simulink model "LF_AC29bus_HVDCdemo_V2_1"  (R2019b)
settings: Solver=FixedStepDiscrete  StartTime=0.0  StopTime=fix(6/Ts)*Ts  FixedStep=Ts  RelTol=1e-3
InitFcn:
  | Ts_avg=150e-6;
  | Ts=50e-6;
  | 
  | %Tc_stab = 1/60/5;
  | %Tc_stab = 2/60;
  | Tc_stab = Ts;
  | 
  | 
  | Ts_avg=150e-6;
  | 
  | Ts=50e-6;
  | 
  | % Rectifier AC side :
  | VLL_nom_R = 735e3; % V
  | Fnom_R = 60;           % Hz
  | 
  | % Inverter AC side :
  | VLL_nom_I = 735e3; % V
  | Fnom_I = 60;           % Hz
  | 
  | % DC :
  | Vdc_nom = 500e3;   % V
  | Idc_nom  = 2000;     % A
undefined symbols (not defined in the file): D1, D11, Delta, test_alpha
libraries: powerlib x223, powerlib_meascontrol x57, simulink x22, sps_avr x7
(part 10 of 10)

== system LF_AC29bus_HVDCdemo_V2_1/HVDC_network_avg/Rectifier Control and Protection (Average model)/Rectifier Pole Control (Current)/Gamma Regulator/PI Regulator with external limits and linrarized Kp (Discrete)1/S16 ==
  note: INTEGRATOR with External limits & Reset & Hold
  note: Gain * Ts
  Max : Inport
  Min : Inport  Port=2
  In : Inport  Port=3
  Reset : Inport  Port=4
  Hold : Inport  Port=5
  Reset Value : Inport  Port=6
  Gain1 : Gain  Gain=k*st  SaturateOnIntegerOverflow=on  OutDataTypeStr=Inherit: Same as input  ParamDataTypeStr=Inherit: Same as input
  IC = ic : UnitDelay  InitialCondition=ic  SampleTime=st  HasFrameUpgradeWarning=on
  Logical Operator4 : Logic  Operator=OR
  MinMax : MinMax  Inputs=2  SaturateOnIntegerOverflow=on  InputSameDT=on
  MinMax1 : MinMax  Function=max  Inputs=2  SaturateOnIntegerOverflow=on  InputSameDT=on
  Saturation Dynamic : simulink/Discontinuities/Saturation Dynamic  OutMin=[]  OutMax=[]  OutDataTypeStr=Inherit: Same as second input  OutDataType=fixdt(1, 16)  OutScaling=2^-10  DoSatur=off
  Sum : Sum  SaturateOnIntegerOverflow=on  InputSameDT=on  OutDataTypeStr=Inherit: Same as first input
  Switch2 : Switch  Criteria=u2 > Threshold  SaturateOnIntegerOverflow=on  InputSameDT=on
  Switch3 : Switch  Criteria=u2 > Threshold  SaturateOnIntegerOverflow=on  InputSameDT=on
  Switch7 : Switch  Criteria=u2 > Threshold  SaturateOnIntegerOverflow=on  InputSameDT=on
  Out : Outport  InitialOutput=0
  wires:
  Saturation Dynamic/1 -> Out/1, IC = ic/1
  Gain1/1 -> Sum/1
  In/1 -> Gain1/1
  Sum/1 -> Saturation Dynamic/2
  Hold/1 -> Logical Operator4/1
  Reset/1 -> Switch7/2, Logical Operator4/2
  Logical Operator4/1 -> Switch2/2, Switch3/2
  Switch2/1 -> MinMax/1
  Max/1 -> Switch2/3, MinMax/2
  Reset Value/1 -> Switch7/1
  MinMax/1 -> Saturation Dynamic/1
  MinMax1/1 -> Saturation Dynamic/3
  Switch3/1 -> MinMax1/1
  Min/1 -> Switch3/3, MinMax1/2
  IC = ic/1 -> Switch7/3
  Switch7/1 -> Switch3/1, Sum/2, Switch2/1

== system LF_AC29bus_HVDCdemo_V2_1/HVDC_network_avg/Rectifier Control and Protection (Average model)/Rectifier Pole Control (Current)/Voltage Regulator/PI Regulator with external limits and linrarized Kp (Discrete)/Kp Linearisation ==
  note: Kp Linearization
  Alpha_lin : Inport
  Kp : Inport  Port=2
  Inv : Inport  Port=3
  Min_lin : Inport  Port=4
  Max_lin : Inport  Port=5
  Constant3 : Constant  Value=On_lin
  Data Type Conversion : DataTypeConversion  OutDataTypeStr=boolean  SaturateOnIntegerOverflow=on  RndMeth=Zero
  Logical Operator : Logic  Operator=NOT
  Logical Operator1 : Logic  Operator=NOT
  Math Function : Math  Operator=reciprocal  SaturateOnIntegerOverflow=on
  Prod2 : Product  Inputs=3  SaturateOnIntegerOverflow=on  InputSameDT=on  OutDataTypeStr=Inherit: Same as first input
  Saturation Dynamic : simulink/Discontinuities/Saturation Dynamic  OutMin=[]  OutMax=[]  OutDataTypeStr=Inherit: Same as second input  OutDataType=fixdt(1, 16)  OutScaling=2^-10  DoSatur=off
  Switch : Switch  Criteria=u2 > Threshold  SaturateOnIntegerOverflow=on  InputSameDT=on
  Switch1 : Switch  Criteria=u2 > Threshold  SaturateOnIntegerOverflow=on  InputSameDT=on
  Trigonometric Function : Trigonometry
  Trigonometric Function1 : Trigonometry
  k : Gain  Gain=pi/180  SaturateOnIntegerOverflow=on  OutDataTypeStr=Inherit: Same as input  ParamDataTypeStr=Inherit: Same as input
  k1 : Gain  Gain=pi/180  SaturateOnIntegerOverflow=on  OutDataTypeStr=Inherit: Same as input  ParamDataTypeStr=Inherit: Same as input
  Kp_lin : Outport  InitialOutput=0
  wires:
  Min_lin/1 -> Switch/1, Saturation Dynamic/3
  Max_lin/1 -> Saturation Dynamic/1, Switch/3
  Alpha_lin/1 -> Saturation Dynamic/2
  Math Function/1 -> Prod2/2
  Trigonometric Function1/1 -> Math Function/1
  k/1 -> Trigonometric Function1/1
  Kp/1 -> Switch1/1, Prod2/3
  Inv/1 -> Logical Operator/1
  Logical Operator/1 -> Switch/2
  Trigonometric Function/1 -> Prod2/1
  Saturation Dynamic/1 -> k/1
  k1/1 -> Trigonometric Function/1
  Switch/1 -> k1/1
  Switch1/1 -> Kp_lin/1
  Prod2/1 -> Switch1/3
  Logical Operator1/1 -> Switch1/2  "off"
  Constant3/1 -> Data Type Conversion/1
  Data Type Conversion/1 -> Logical Operator1/1

== system LF_AC29bus_HVDCdemo_V2_1/HVDC_network_avg/Rectifier Control and Protection (Average model)/Rectifier Pole Control (Current)/Voltage Regulator/PI Regulator with external limits and linrarized Kp (Discrete)/S16 ==
  note: INTEGRATOR with External limits & Reset & Hold
  note: Gain * Ts
  Max : Inport
  Min : Inport  Port=2
  In : Inport  Port=3
  Reset : Inport  Port=4
  Hold : Inport  Port=5
  Reset Value : Inport  Port=6
  Gain1 : Gain  Gain=k*st  SaturateOnIntegerOverflow=on  OutDataTypeStr=Inherit: Same as input  ParamDataTypeStr=Inherit: Same as input
  IC = ic : UnitDelay  InitialCondition=ic  SampleTime=st  HasFrameUpgradeWarning=on
  Logical Operator4 : Logic  Operator=OR
  MinMax : MinMax  Inputs=2  SaturateOnIntegerOverflow=on  InputSameDT=on
  MinMax1 : MinMax  Function=max  Inputs=2  SaturateOnIntegerOverflow=on  InputSameDT=on
  Saturation Dynamic : simulink/Discontinuities/Saturation Dynamic  OutMin=[]  OutMax=[]  OutDataTypeStr=Inherit: Same as second input  OutDataType=fixdt(1, 16)  OutScaling=2^-10  DoSatur=off
  Sum : Sum  SaturateOnIntegerOverflow=on  InputSameDT=on  OutDataTypeStr=Inherit: Same as first input
  Switch2 : Switch  Criteria=u2 > Threshold  SaturateOnIntegerOverflow=on  InputSameDT=on
  Switch3 : Switch  Criteria=u2 > Threshold  SaturateOnIntegerOverflow=on  InputSameDT=on
  Switch7 : Switch  Criteria=u2 > Threshold  SaturateOnIntegerOverflow=on  InputSameDT=on
  Out : Outport  InitialOutput=0
  wires:
  Saturation Dynamic/1 -> Out/1, IC = ic/1
  Gain1/1 -> Sum/1
  In/1 -> Gain1/1
  Sum/1 -> Saturation Dynamic/2
  Hold/1 -> Logical Operator4/1
  Reset/1 -> Switch7/2, Logical Operator4/2
  Logical Operator4/1 -> Switch2/2, Switch3/2
  Switch2/1 -> MinMax/1
  Max/1 -> Switch2/3, MinMax/2
  Reset Value/1 -> Switch7/1
  MinMax/1 -> Saturation Dynamic/1
  MinMax1/1 -> Saturation Dynamic/3
  Switch3/1 -> MinMax1/1
  Min/1 -> Switch3/3, MinMax1/2
  IC = ic/1 -> Switch7/3
  Switch7/1 -> Switch3/1, Sum/2, Switch2/1

== matlab function LF_AC29bus_HVDCdemo_V2_1/HVDC_network_avg/Inverter Average model/HVDC_CONV_AVG/Average Model Computation/DC_AVG_EQ MATLAB Function ==
  data: Ud output; alpha_deg input; Tap_pu input; Id input; I_dq output; Udi0 input; w input; Lc parameter size=1; m output; R12 parameter size=1; Vf parameter size=1; Ron parameter size=1; Ratio_nom parameter size=1
% Embedded function : DC_AVG_EQ
% By: Silvano Casoria (Hydro-Queec)
% Date: January 2011, December 2012
% Description: Implement the equations of the average model of an HVDC
%              converter unit (transformer and 6 pulse bridge).
% 
%
function [Ud,I_dq, m]=DC_AVG_EQ(alpha_deg,Tap_pu,Id,Udi0,w,...
Lc, R12, Vf, Ron, Ratio_nom)
%
% INPUTS:
% alpha_deg: Firing angle from the control system (deg)
% Tap_pu: Per-unit tap ratio (Npripary/Nsecondary)
% Id:   DC current (A)
% Udi0: Ideal no load direct voltage (V)
% w:    System angular frequency (rad/s)
%
% OUTPUTS:
% Ud: Direct voltage (V)
% I_dq: Two element vector [I_d, I_q] with I_d = d axis component of the
%       fondamental primary phase current, I_q = q axis componenet.
% m : Four element vector to measure internal variables.
%
% PARAMETERS (for one 6p bridge. Calculated in the model mask):
% Lc  = Commutation inductance, seen from the secondary (H)
% R12 = Total transformer resistance, seen from the secondary (ohm)
% Vf  = Thristor/Diode forward voltage (V)
% Ron = Thristor/Diode On resistance (ohm)
% Ratio_nom = Nominal transformer ratio (Uprim/Usec)

% Initialisation and declaration:
m = [0 0 0 0];

% Xc calculation :
Xc = Lc * w;

% Intermediary calculation :
Rc = Xc * 3/pi;              % Commutation resistance Rc (ohm)
Cos_alpha = cosd(alpha_deg); % (rad)
 
% Overlap angle calculation :
mu_deg = acosd( LIM((Cos_alpha-2*(Rc*Id/LIM(Udi0,eps,1e6))),-1,1) )- ...
         alpha_deg;  %(deg)
mu  = mu_deg*1.745329e-2;    % (rad)

% Exctinctoin angle (gamma_deg) deduction :
gamma_deg = 180 - alpha_deg - mu_deg;

% Transformer windings & Thyristor resistance drop Mean value
% a functoin of the commutation interval:
Req      = (2 - mu_deg/120) * (R12+Ron);
Req_drop = Req * Id;

% Thyristors forward drop:
Thy_drop = 2*Vf;

% Ud calculation :
Ud  = Udi0 * Cos_alpha - Rc*Id - Req_drop - Thy_drop;

% Fondamental primary phase current Ia1 components d and q axis 
% (Ia1 = I_d + j*I_q) (rms values):
Den = (Tap_pu*Ratio_nom*Xc*4*sqrt(6));
I_d = Udi0*(cosd(2*alpha_deg)-cosd(2*mu_deg+2*alpha_deg))/Den;
I_q = -Udi0*(2*mu+sind(2*alpha_deg) - sind(2*mu_deg+2*alpha_deg))/Den;
I_dq = [I_d, I_q]';
   
% Reactive power consumption (always positive):
Q = -(I_q*Udi0*pi*Ratio_nom*Tap_pu)/sqrt(6);  % (var)

% Active AC power flowing into the converter transformer :
P = (I_d*Udi0*pi*Ratio_nom*Tap_pu)/sqrt(6);   % (W)

% Measurements:
m(1) = Q;
m(2) = mu_deg;
m(3) = gamma_deg;
m(4) = P;

% ----------
function [Y_lim] = LIM(Y,Min,Max)
% Description : The output is the input signal limited between the
%               values Min and Max ([Min,Max]).
if (Y >= Max)
    Y_lim = Max;
elseif (Y <= Min)
    Y_lim = Min;
else
    Y_lim = Y;
end
% ======================= E N D ===============================

== matlab function LF_AC29bus_HVDCdemo_V2_1/HVDC_network_avg/Rectifier Average model/HVDC_CONV_AVG/Average Model Computation/DC_AVG_EQ MATLAB Function ==
  data: Ud output; alpha_deg input; Tap_pu input; Id input; I_dq output; Udi0 input; w input; Lc parameter size=1; m output; R12 parameter size=1; Vf parameter size=1; Ron parameter size=1; Ratio_nom parameter size=1
% Embedded function : DC_AVG_EQ
% By: Silvano Casoria (Hydro-Queec)
% Date: January 2011, December 2012
% Description: Implement the equations of the average model of an HVDC
%              converter unit (transformer and 6 pulse bridge).
% 
%
function [Ud,I_dq, m]=DC_AVG_EQ(alpha_deg,Tap_pu,Id,Udi0,w,...
Lc, R12, Vf, Ron, Ratio_nom)
%
% INPUTS:
% alpha_deg: Firing angle from the control system (deg)
% Tap_pu: Per-unit tap ratio (Npripary/Nsecondary)
% Id:   DC current (A)
% Udi0: Ideal no load direct voltage (V)
% w:    System angular frequency (rad/s)
%
% OUTPUTS:
% Ud: Direct voltage (V)
% I_dq: Two element vector [I_d, I_q] with I_d = d axis component of the
%       fondamental primary phase current, I_q = q axis componenet.
% m : Four element vector to measure internal variables.
%
% PARAMETERS (for one 6p bridge. Calculated in the model mask):
% Lc  = Commutation inductance, seen from the secondary (H)
% R12 = Total transformer resistance, seen from the secondary (ohm)
% Vf  = Thristor/Diode forward voltage (V)
% Ron = Thristor/Diode On resistance (ohm)
% Ratio_nom = Nominal transformer ratio (Uprim/Usec)

% Initialisation and declaration:
m = [0 0 0 0];

% Xc calculation :
Xc = Lc * w;

% Intermediary calculation :
Rc = Xc * 3/pi;              % Commutation resistance Rc (ohm)
Cos_alpha = cosd(alpha_deg); % (rad)
 
% Overlap angle calculation :
mu_deg = acosd( LIM((Cos_alpha-2*(Rc*Id/LIM(Udi0,eps,1e6))),-1,1) )- ...
         alpha_deg;  %(deg)
mu  = mu_deg*1.745329e-2;    % (rad)

% Exctinctoin angle (gamma_deg) deduction :
gamma_deg = 180 - alpha_deg - mu_deg;

% Transformer windings & Thyristor resistance drop Mean value
% a functoin of the commutation interval:
Req      = (2 - mu_deg/120) * (R12+Ron);
Req_drop = Req * Id;

% Thyristors forward drop:
Thy_drop = 2*Vf;

% Ud calculation :
Ud  = Udi0 * Cos_alpha - Rc*Id - Req_drop - Thy_drop;

% Fondamental primary phase current Ia1 components d and q axis 
% (Ia1 = I_d + j*I_q) (rms values):
Den = (Tap_pu*Ratio_nom*Xc*4*sqrt(6));
I_d = Udi0*(cosd(2*alpha_deg)-cosd(2*mu_deg+2*alpha_deg))/Den;
I_q = -Udi0*(2*mu+sind(2*alpha_deg) - sind(2*mu_deg+2*alpha_deg))/Den;
I_dq = [I_d, I_q]';
   
% Reactive power consumption (always positive):
Q = -(I_q*Udi0*pi*Ratio_nom*Tap_pu)/sqrt(6);  % (var)

% Active AC power flowing into the converter transformer :
P = (I_d*Udi0*pi*Ratio_nom*Tap_pu)/sqrt(6);   % (W)

% Measurements:
m(1) = Q;
m(2) = mu_deg;
m(3) = gamma_deg;
m(4) = P;

% ----------
function [Y_lim] = LIM(Y,Min,Max)
% Description : The output is the input signal limited between the
%               values Min and Max ([Min,Max]).
if (Y >= Max)
    Y_lim = Max;
elseif (Y <= Min)
    Y_lim = Min;
else
    Y_lim = Y;
end
% ======================= E N D ===============================
